simulink model "rtwdemo_structsignal2"  (Simulink 7.1)
settings: Solver=FixedStepDiscrete  StartTime=0.0  StopTime=10.0  RelTol=1e-3
PostLoadFcn:
  | load structsignal2.mat;
settings Model: Creator=ajayaram  LastModifiedBy=ajayaram
settings SolverCC: AutoInsertRateTranBlk=on
settings DataIOCC: SaveOutput=off  SaveTime=off
settings OptimizationCC: InlineParams=on  InlineInvariantSignals=on  EnforceIntegerDowncast=off  StateBitsets=on  DataBitsets=on  UseTempVars=on  OptimizeModelRefInitCode=on  LifeSpan=1
settings RTWCC: SystemTargetFile=ert.tlc  GenCodeOnly=on  GenerateMakefile=off  TemplateMakefile=ert_default_tmf  Description=Real-Time Workshop Embedded Coder (no auto configuration)  GenerateReport=on  RTWVerbose=off  ProcessScript=ert_make_rtw_hook  IncludeHyperlinkInReport=on  LaunchReport=on
settings CodeAppCC: IgnoreCustomStorageClasses=off  CustomSymbolStrGlobalVar=rt$N$M  CustomSymbolStrType=$N$M  CustomSymbolStrFcn=$N$M$F  CustomSymbolStrMacro=$N$M
settings ERTTargetCC: GenerateSampleERTMain=on  SuppressErrorStatus=on  SupportAbsoluteTime=off  SupportNonFinite=off  SupportComplex=off  InlinedParameterPlacement=NonHierarchical  RootIOFormat=Structure reference  ERTCustomFileTemplate=example_file_process.tlc

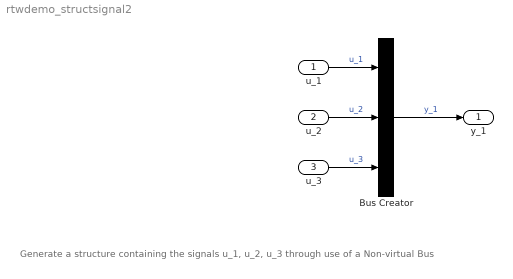
== system rtwdemo_structsignal2 ==
  note: Generate a structure containing the signals
      | u_1, u_2, u_3 through use of a Non-virtual Bus
  u_1 : Inport  OutDataType=sfix(16)  OutScaling=2^0
  u_2 : Inport  Port=2  OutDataType=sfix(16)  OutScaling=2^0
  u_3 : Inport  Port=3  OutDataType=sfix(16)  OutScaling=2^0
  Bus Creator : BusCreator  Inputs=3  UseBusObject=on  NonVirtualBus=on
      settings: AttributesFormatString=%<BlockDescription>  BusObject=MySignals
  y_1 : Outport  OutDataType=sfix(16)  OutScaling=2^0
  wires:
  u_1/1 -> Bus Creator/1  "u_1"
  u_2/1 -> Bus Creator/2  "u_2"
  u_3/1 -> Bus Creator/3  "u_3"
  Bus Creator/1 -> y_1/1  "y_1"
